simulink model "CTRL_LO_ST1_WHFSUM_test"  (R2023b)
settings: Solver=VariableStepAuto  StartTime=0.0  StopTime=10.0  RelTol=1e-3
libraries: CTRL_LO_ST1_WHFSUM x1
settings Model: Creator=blatak  LastModifiedBy=blatak

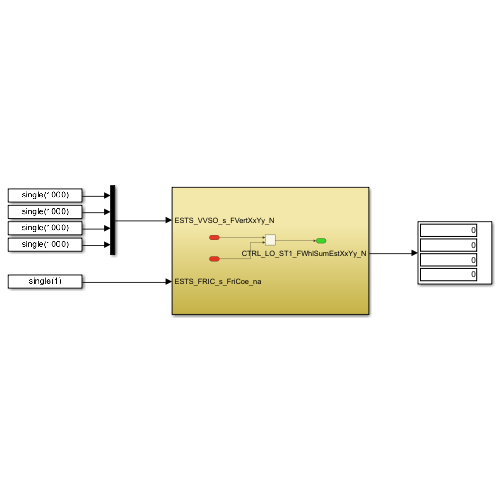
[thumbnail: Simulink's stored preview of the top-level diagram]
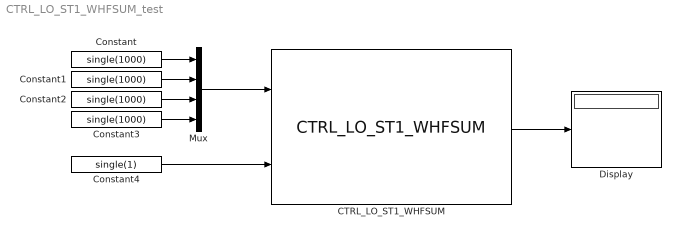
== system CTRL_LO_ST1_WHFSUM_test ==
  CTRL_LO_ST1_WHFSUM : CTRL_LO_ST1_WHFSUM/CTRL_LO_ST1_WHFSUM  SystemSampleTime=-1  VariantActivationTime=update diagram  AllowFlexibleInterface=on  Latency=0  AutoFrameSizeCalculation=off
  Constant{,1..3} (4 alike) : Constant  Value=single(1000)
  Constant4 : Constant  Value=single(1)
  Display : Display
  Mux : Mux
  wires:
  Constant4/1 -> CTRL_LO_ST1_WHFSUM/2
  Constant/1 -> Mux/1
  Constant1/1 -> Mux/2
  Constant2/1 -> Mux/3
  Constant3/1 -> Mux/4
  Mux/1 -> CTRL_LO_ST1_WHFSUM/1
  CTRL_LO_ST1_WHFSUM/1 -> Display/1
